simulink model "Trajectory_Tracking_Car_NonLin_MPC"  (R2022b)
settings: Solver=FixedStepAuto  StartTime=0.0  StopTime=63  FixedStep=Ts  RelTol=1e-3
values from neighbouring files (symbols this model uses):
  alpha = 3    [Setup_Trajectory_FL_MPC.m]    (also in Setup_trajectory_Backstepping.m; Setup_trajectory_NL_MPC.m)
  beta = 1.7    [Setup_Trajectory_FL_MPC.m]    (also in Setup_trajectory_Backstepping.m; Setup_trajectory_NL_MPC.m)
  l = 0.256    [Setup_Trajectory_FL_MPC.m]    (also in Setup_trajectory_Backstepping.m; Setup_trajectory_NL_MPC.m)
  N = 10    [Setup_Trajectory_FL_MPC.m]    (also in Setup_trajectory_Backstepping.m; Setup_trajectory_NL_MPC.m = 5)
  q0 = [x0;y0;theta0;phi0]    [Setup_Trajectory_FL_MPC.m]    (also in Setup_trajectory_Backstepping.m; Setup_trajectory_NL_MPC.m)
  qu = 0.00001    (= 1e-05)    [Setup_Trajectory_FL_MPC.m]    (also in Setup_trajectory_NL_MPC.m = 0.0001)
  qz = 10    [Setup_Trajectory_FL_MPC.m]    (also in Setup_trajectory_NL_MPC.m = 1)
  thetar = unwrap(atan2(ydr./v1r,xdr./v1r))    [Setup_Trajectory_FL_MPC.m]    (also in Setup_trajectory_Backstepping.m; Setup_trajectory_NL_MPC.m)
  Ts = 0.01    [Setup_Trajectory_FL_MPC.m]    (also in Setup_trajectory_Backstepping.m; Setup_trajectory_NL_MPC.m = 0.1)
  v1max = 2    [Setup_Trajectory_FL_MPC.m]    (also in Setup_trajectory_Backstepping.m; Setup_trajectory_NL_MPC.m)
  v2max = 2    [Setup_Trajectory_FL_MPC.m]    (also in Setup_trajectory_Backstepping.m = 10; Setup_trajectory_NL_MPC.m)
settings Model: Creator=cricr  LastModifiedBy=user
settings SolverCC: AlgebraicLoopSolver=TrustRegion
settings DataIOCC: ReturnWorkspaceOutputs=off
settings DebuggingCC: UnconnectedInputMsg=warning  UnconnectedOutputMsg=warning  UnconnectedLineMsg=warning  SFMachineParentedDataDiag=warning  ArithmeticOperatorsInVariantConditions=warning
settings ModelReferenceCC: EnableRefExpFcnMdlSchedulingChecks=on
settings SFSimCC: SimUseLocalCustomCode=off  CustomCodeUndefinedFunction=UseInterfaceOnly
settings RTWCC: RTWUseLocalCustomCode=off

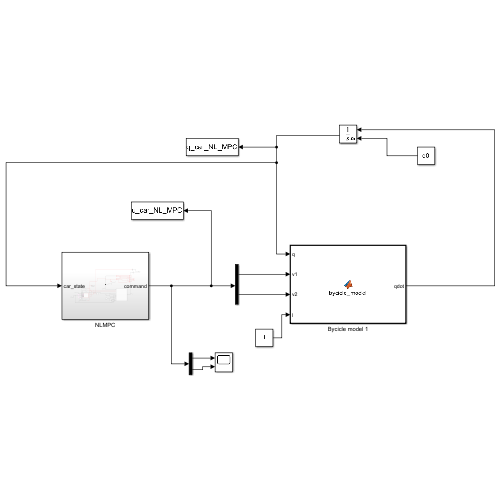
[thumbnail: Simulink's stored preview of the top-level diagram]
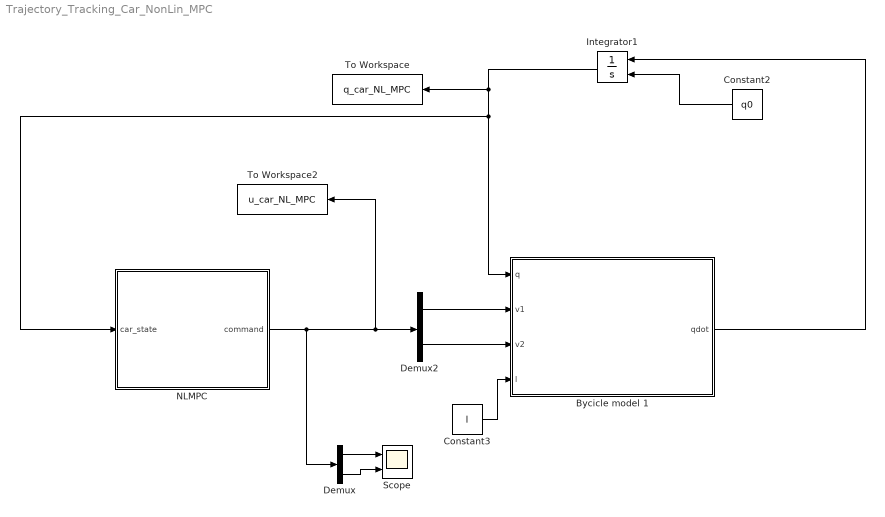
== system Trajectory_Tracking_Car_NonLin_MPC ==
  Bycicle model 1 : MATLAB Function  TreatAsAtomicUnit=on
  Constant2 : Constant  Value=q0
  Constant3 : Constant  Value=l
  Demux : Demux  Outputs=2
  Demux2 : Demux  Outputs=2
  Integrator1 : Integrator  InitialConditionSource=external
  NLMPC : Subsystem
  Scope : Scope  NumInputPorts=2
  To Workspace : ToWorkspace  VariableName=q_car_NL_MPC  SaveFormat=Timeseries  SampleTime=-1
  To Workspace2 : ToWorkspace  VariableName=u_car_NL_MPC  SaveFormat=Timeseries  SampleTime=-1
  wires:
  Constant2/1 -> Integrator1/2
  Bycicle model 1/1(qdot) -> Integrator1/1
  Demux2/1 -> Bycicle model 1/2(v1)
  Demux2/2 -> Bycicle model 1/3(v2)
  Constant3/1 -> Bycicle model 1/4(l)
  Integrator1/1 -> To Workspace/1, NLMPC/1(car_state), Bycicle model 1/1(q)
  Demux/1 -> Scope/1
  Demux/2 -> Scope/2
  NLMPC/1(command) -> Demux/1, To Workspace2/1, Demux2/1

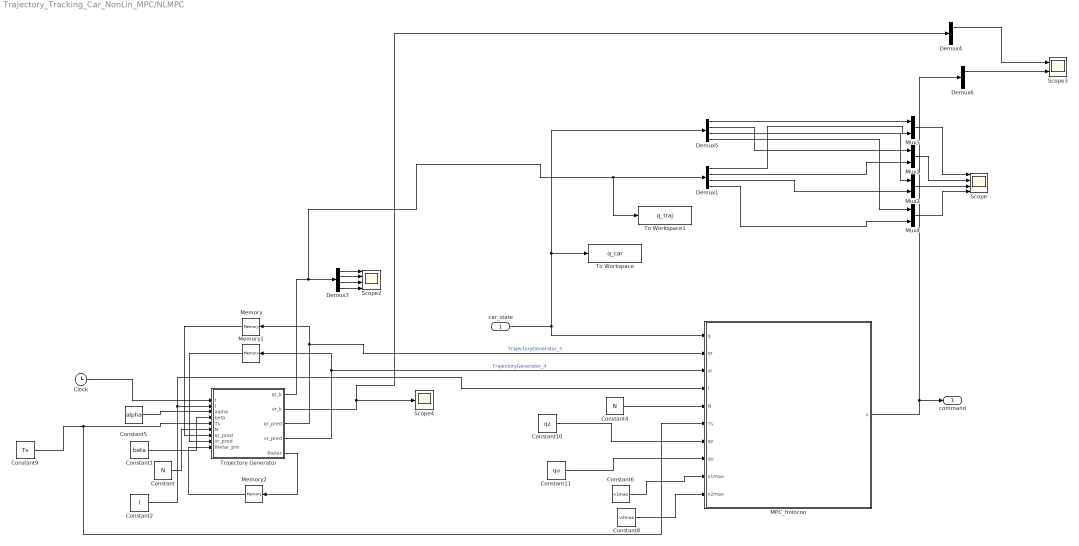
== system Trajectory_Tracking_Car_NonLin_MPC/NLMPC ==
  car_state : Inport
  Clock : Clock
  Constant : Constant  Value=N
  Constant1 : Constant  Value=beta
  Constant10 : Constant  Value=qz
  Constant11 : Constant  Value=qu
  Constant2 : Constant  Value=l
  Constant4 : Constant  Value=N
  Constant5 : Constant  Value=alpha
  Constant6 : Constant  Value=v1max
  Constant8 : Constant  Value=v2max
  Constant9 : Constant  Value=Ts
  Demux1 : Demux
  Demux3 : Demux
  Demux4 : Demux  Outputs=2
  Demux5 : Demux
  Demux6 : Demux  Outputs=2
  MPC_fmincon : MATLAB Function  TreatAsAtomicUnit=on
  Memory : Memory  InitialCondition=zeros(4,N)
  Memory1 : Memory  InitialCondition=zeros(2,N)
  Memory2 : Memory  InitialCondition=thetar(1)
  Mux{1..4} (4 alike) : Mux  Inputs=2
  Scope : Scope  NumInputPorts=4
  Scope2 : Scope  NumInputPorts=4
  Scope3 : Scope  NumInputPorts=2
  Scope4 : Scope
  To Workspace : ToWorkspace  VariableName=q_car  SaveFormat=Timeseries  SampleTime=-1
  To Workspace1 : ToWorkspace  VariableName=q_traj  SaveFormat=Timeseries  SampleTime=-1
  Trajectory Generator : MATLAB Function  TreatAsAtomicUnit=on
  command : Outport
  wires:
  Demux5/2 -> Mux1/1
  Demux6/1 -> Scope3/2
  Demux5/4 -> Mux4/1
  Mux2/1 -> Scope/3
  Mux3/1 -> Scope/1
  Constant5/1 -> Trajectory Generator/3(alpha)
  Demux3/1 -> Scope2/1
  Constant9/1 -> Trajectory Generator/5(Ts), MPC_fmincon/6(Ts)
  Trajectory Generator/1(qr_k) -> Demux3/1, To Workspace1/1, Demux1/1
  Trajectory Generator/2(vr_k) -> Scope4/1, Demux4/1
  Demux4/1 -> Scope3/1
  Demux1/3 -> Mux2/2
  Mux1/1 -> Scope/2
  Demux1/4 -> Mux4/2
  Clock/1 -> Trajectory Generator/1(t)
  Mux4/1 -> Scope/4
  Demux3/2 -> Scope2/2
  Demux5/1 -> Mux3/1
  Demux3/4 -> Scope2/4
  Constant1/1 -> Trajectory Generator/4(beta)
  car_state/1 -> MPC_fmincon/1(q), To Workspace/1, Demux5/1
  Constant8/1 -> MPC_fmincon/10(v2max)
  Demux1/1 -> Mux3/2
  MPC_fmincon/1(v) -> Demux6/1, command/1
  Constant2/1 -> MPC_fmincon/4(l), Trajectory Generator/2(l)
  Demux1/2 -> Mux1/2
  Demux5/3 -> Mux2/1
  Demux3/3 -> Scope2/3
  Trajectory Generator/3(qr_pred) -> Memory/1, MPC_fmincon/2(qr)  "TrajectoryGenerator_3"
  Trajectory Generator/4(vr_pred) -> Memory1/1, MPC_fmincon/3(vr)  "TrajectoryGenerator_4"
  Constant/1 -> Trajectory Generator/6(N)
  Memory/1 -> Trajectory Generator/7("qr_pred ")
  Memory1/1 -> Trajectory Generator/8("vr_pred ")
  Constant4/1 -> MPC_fmincon/5(N)
  Constant10/1 -> MPC_fmincon/7(qz)
  Constant11/1 -> MPC_fmincon/8(qu)
  Constant6/1 -> MPC_fmincon/9(v1max)
  Memory2/1 -> Trajectory Generator/9(thetar_pre)
  Trajectory Generator/5(thetar) -> Memory2/1

== matlab function Trajectory_Tracking_Car_NonLin_MPC/NLMPC/MPC_fmincon ==
  data: q input; v output; qr input; vr input; l input; N input; Ts input; qz input; qu input; v1max input; v2max input
function v= MPC_fmincon_tracking_controller(q,qr,vr,l,N,Ts,qz,qu,v1max,v2max)


Qhat=qz*eye(4*N);
Rhat=qu*eye(2*N);






%Set theoretic MPC online optimization


    function obj=obj_fun(u,q,qr,vr,l,Ts,Qhat,Rhat,N)


        %         qtilde=zeros(4*N,1);
        %
        %         qtilde(1:4,1)=q-qr(:,1);
        %
        %         qcurr=q;
        %
        %         for i=1:N-1
        %
        %
        %             qnext = qcurr +Ts*[cos(qcurr(3)) 0;
        %                 sin(qcurr(3)) 0;
        %                 tan(qcurr(4))/l 0;
        %                 0          1]*u(2*i-1:2*i);
        %
        %             qtilde(4*i+1:4*i+4,1)=qnext-qr(:,i+1);
        %
        %             qcurr=qnext;
        %
        %         end




        qtilde=zeros(4*N,1);

        qcurr=q;

        for i=1:N


            qnext = qcurr +Ts*[cos(qcurr(3)) 0;
                sin(qcurr(3)) 0;
                tan(qcurr(4))/l 0;
                0          1]*u(2*i-1:2*i);

            qtilde(4*i-3:4*i,1)=qnext-qr(:,i);

            qcurr=qnext;

        end





        Wr=[];

        for j=1:N
            Wr=[Wr; vr(:,j)];
        end

        obj=qtilde'*Qhat*qtilde+(u-Wr)'*Rhat*(u-Wr);


    end







T=[-1 0; 0 -1; 1 0; 0 1];
% Hk=T/T_FL;
g=[v1max;v2max;v1max;v2max];



 H_constr=zeros(4*N,2*N);
 g_constr=zeros(4*N,1);

 for k=1:N

     H_constr(4*k-3:4*k,2*k-1:2*k)=T;
     g_constr(4*k-3:4*k,1)=g;

 end




options=optimoptions('fmincon','Display','off','Algorithm','sqp');

options.MaxIterations = 100;
options.ConstraintTolerance = 1.0e-6;
options.OptimalityTolerance = 1.0e-6;



usol = fmincon(@(u)obj_fun(u,q,qr,vr,l,Ts,Qhat,Rhat,N),zeros(2*N,1),H_constr,g_constr,[],[],[],[],[],options);
v=usol(1:2);



end

== matlab function Trajectory_Tracking_Car_NonLin_MPC/NLMPC/Trajectory Generator ==
  data: t input; qr_k output; vr_k output; l input; alpha input; beta input; Ts input; qr_pred output size=[4 N]; vr_pred output size=[2 N]; N input; qr_pred input; vr_pred input; thetar_pre input; thetar output
function [qr_k,vr_k,qr_pred, vr_pred,thetar] = Trajectory(t,l,alpha,beta,Ts,N,qr_pred,vr_pred,thetar_pre)




xr=alpha*sin(t/beta);
yr=alpha*sin(t/(2*beta));

xdr=alpha*cos(t/beta)*(1/(beta));
ydr=alpha*cos(t/(2*beta))*(1/(2*beta));


xddr=-alpha*sin(t/beta)*(1/(beta))^2;
yddr=-alpha*sin(t/(2*beta))*(1/(2*beta))^2;

xdddr=-alpha*cos(t/beta)*(1/(beta))^3;
ydddr=-alpha*cos(t/(2*beta))*(1/(2*beta))^3;

%Driving velocity reference
v1r=sqrt(xdr^2+ydr^2); %Linear velocity of the trajectory


thetar=atan2(ydr/v1r,xdr/v1r);

theta=[thetar_pre thetar];

theta=unwrap(theta);
thetar=theta(2);


%Steering angle reference
phir=atan(l*(yddr*xdr-xddr*ydr)/v1r^3);

%Steering velocity reference
v2r=l*v1r*((ydddr*xdr-xdddr*ydr)*v1r^2-3*(yddr*xdr-xddr*ydr)*(xdr*xddr+ydr*yddr))/(v1r^6+l^2*(yddr*xdr-xddr*ydr)^2);


qr_k=[xr;yr;thetar;phir];
vr_k=[v1r;v2r];


for i=1:N
    t=t+(i-1)*Ts;
    xr=alpha*sin(t/beta);
    yr=alpha*sin(t/(2*beta));

    xdr=alpha*cos(t/beta)*(1/(beta));
    ydr=alpha*cos(t/(2*beta))*(1/(2*beta));


    xddr=-alpha*sin(t/beta)*(1/(beta))^2;
    yddr=-alpha*sin(t/(2*beta))*(1/(2*beta))^2;

    xdddr=-alpha*cos(t/beta)*(1/(beta))^3;
    ydddr=-alpha*cos(t/(2*beta))*(1/(2*beta))^3;



    %Driving velocity reference
    v1r=sqrt(xdr^2+ydr^2); %Linear velocity of the trajectory

    

    thetar=atan2(ydr/v1r,xdr/v1r);

    if i==1
        theta=[thetar_pre thetar];
        theta=unwrap(theta);
        thetar=theta(2);
        thetar_pre=thetar;

    else
       
        theta=[thetar_pre thetar];
        theta=unwrap(theta);
        thetar=theta(2);


    end


    %Steering angle reference
    phir=atan(l*(yddr*xdr-xddr*ydr)/v1r^3);

    %Steering velocity reference
    v2r=l*v1r*((ydddr*xdr-xdddr*ydr)*v1r^2-3*(yddr*xdr-xddr*ydr)*(xdr*xddr+ydr*yddr))/(v1r^6+l^2*(yddr*xdr-xddr*ydr)^2);



    %Nonlinear model reference state
    qr_pred(:,i)=[xr;yr;thetar;phir];
    vr_pred(:,i)=[v1r;v2r];

end

 qr_pred(3,:)= unwrap(qr_pred(3,:));

== matlab function Trajectory_Tracking_Car_NonLin_MPC/Bycicle model 1 ==
  data: q input; qdot output; v1 input; v2 input; l input
function qdot  = bycicle_model(q,v1,v2,l)

%This function implements the car kinematic model
x=q(1);
y=q(2);
theta=q(3);
phi=q(4);

q1dot=v1*cos(theta);
q2dot=v1*sin(theta);
q3dot = v1*tan(phi)/l;
q4dot = v2;


qdot= [q1dot;q2dot;q3dot;q4dot];
end
